simulink model "discrete"  (R2023b)
settings: Solver=FixedStepAuto  StartTime=0.0  StopTime=20  FixedStep=0.01  RelTol=1e-3
InitFcn:
  | clc;clear
  | close all
  | g = [0;2.092];
  | k1 = [-141.9203 -4.5243];
  | k2 = [-101.5134 -3.1941];
  | x0 = [0.4;-10];
libraries: simulink x1
settings Model: Creator=IHC  LastModifiedBy=IHC

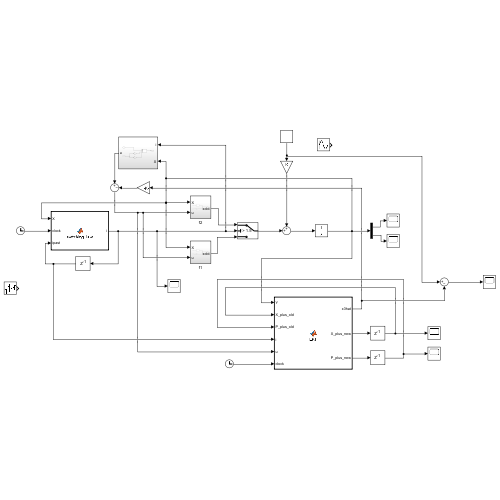
[thumbnail: Simulink's stored preview of the top-level diagram]
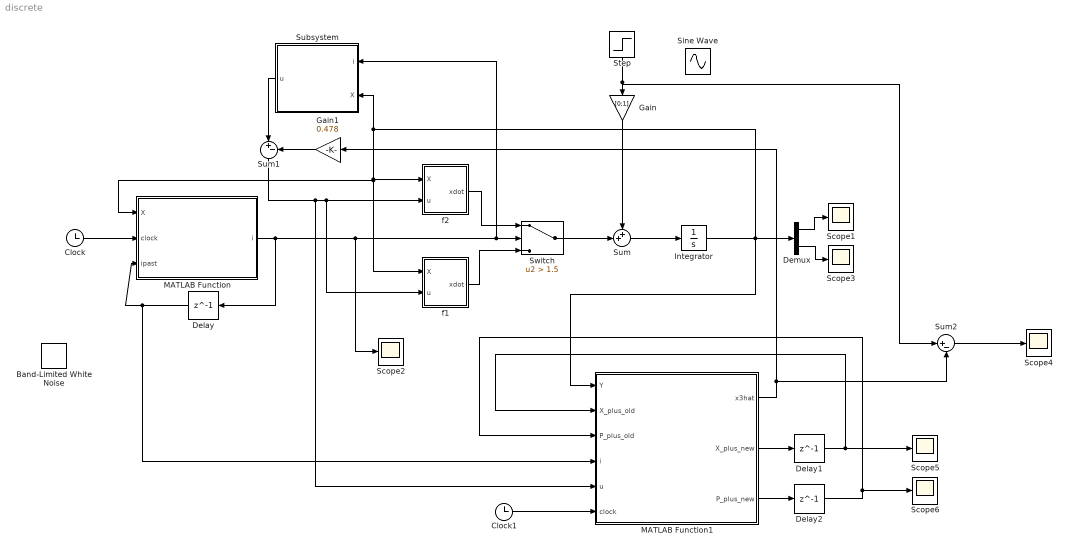
== system discrete ==
  Band-Limited White Noise : simulink/Sources/Band-Limited White Noise  Cov=[0.1]  Ts=0.1  seed=[23341]
  Clock : Clock
  Clock1 : Clock
  Delay : Delay  DelayLength=1  InitialCondition=2
  Delay1 : Delay  DelayLength=1  InitialCondition=[x0;0]
  Delay2 : Delay  DelayLength=1  InitialCondition=diag([0.001;0.001;10])
  Demux : Demux  Outputs=2
  Gain : Gain  Gain=[0;1]
  Gain1 : Gain  Gain=0.478
  Integrator : Integrator  InitialCondition=x0
  MATLAB Function : MATLAB Function  TreatAsAtomicUnit=on
  MATLAB Function1 : MATLAB Function  TreatAsAtomicUnit=on
  Scope{1..6} (6 alike) : Scope
  Sine Wave : Sin  SampleTime=0
  Step : Step  Time=0  SampleTime=0
  Subsystem : Subsystem
  Sum : Sum  Inputs=++|
  Sum1 : Sum  Inputs=|+-
  Sum2 : Sum  Inputs=|+-
  Switch : Switch  Criteria=u2 > Threshold  Threshold=1.5  SaturateOnIntegerOverflow=off  InputSameDT=off
  f1 : Subsystem
  f2 : Subsystem
  wires:
  Clock/1 -> MATLAB Function/2(clock)
  Subsystem/1(u) -> Sum1/1
  Demux/1 -> Scope1/1
  Demux/2 -> Scope3/1
  Delay/1 -> MATLAB Function1/4(i), MATLAB Function/3(ipast)
  MATLAB Function/1(i) -> Delay/1, Scope2/1, Subsystem/1(i), Switch/2
  f2/1(xdot) -> Switch/1
  f1/1(xdot) -> Switch/3
  Switch/1 -> Sum/2
  Sum/1 -> Integrator/1
  Gain/1 -> Sum/1
  Gain1/1 -> Sum1/2
  Step/1 -> Sum2/1, Gain/1
  Integrator/1 -> MATLAB Function1/1(Y), Demux/1, f1/1(X), MATLAB Function/1(X), f2/1(X), Subsystem/2(X)
  Sum1/1 -> MATLAB Function1/5(u), f1/2(u), f2/2(u)
  Clock1/1 -> MATLAB Function1/6(clock)
  MATLAB Function1/2(X_plus_new) -> Delay1/1
  MATLAB Function1/3(P_plus_new) -> Delay2/1
  Delay2/1 -> MATLAB Function1/3(P_plus_old), Scope6/1
  Delay1/1 -> Scope5/1, MATLAB Function1/2(X_plus_old)
  Sum2/1 -> Scope4/1
  MATLAB Function1/1(x3hat) -> Gain1/1, Sum2/2

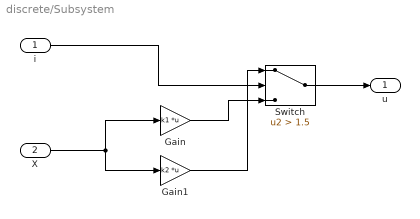
== system discrete/Subsystem ==
  i : Inport
  X : Inport  Port=2
  Gain : Gain  Gain=k1  Multiplication=Matrix(K*u)
  Gain1 : Gain  Gain=k2  Multiplication=Matrix(K*u)
  Switch : Switch  Criteria=u2 > Threshold  Threshold=1.5  SaturateOnIntegerOverflow=off  InputSameDT=off
  u : Outport
  wires:
  Switch/1 -> u/1
  i/1 -> Switch/2
  X/1 -> Gain1/1, Gain/1
  Gain/1 -> Switch/3
  Gain1/1 -> Switch/1

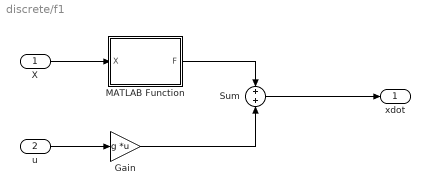
== system discrete/f1 ==
  X : Inport
  u : Inport  Port=2
  Gain : Gain  Gain=g  Multiplication=Matrix(K*u)
  MATLAB Function : MATLAB Function  TreatAsAtomicUnit=on
  Sum : Sum
  xdot : Outport
  wires:
  u/1 -> Gain/1
  X/1 -> MATLAB Function/1(X)
  Gain/1 -> Sum/2
  MATLAB Function/1(F) -> Sum/1
  Sum/1 -> xdot/1

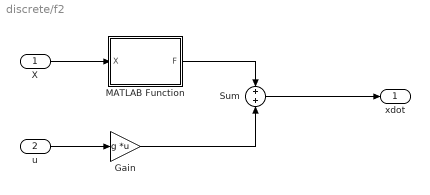
== system discrete/f2 ==
  X : Inport
  u : Inport  Port=2
  Gain : Gain  Gain=g  Multiplication=Matrix(K*u)
  MATLAB Function : MATLAB Function  TreatAsAtomicUnit=on
  Sum : Sum
  xdot : Outport
  wires:
  Sum/1 -> xdot/1
  u/1 -> Gain/1
  MATLAB Function/1(F) -> Sum/1
  Gain/1 -> Sum/2
  X/1 -> MATLAB Function/1(X)

== matlab function discrete/f2/MATLAB Function ==
  data: X input; F output
function F = fcn(X)
x1 = X(1);
x2 = X(2);
alpha = -7.2*10^10*(x1+0.5)*exp(-8750/(x2+350))+0.5;
beta = 1.506*10^13*(x1+0.5)*exp(-8750/(x2+350))-104.6;
f1=-2*x1+alpha;
f2 =-4.092*x2+beta;
F=[f1;f2];
end

== matlab function discrete/f1/MATLAB Function ==
  data: X input; F output
function F = fcn(X)
x1 = X(1);
x2 = X(2);
alpha = -7.2*10^10*(x1+0.5)*exp(-8750/(x2+350))+0.5;
beta = 1.506*10^13*(x1+0.5)*exp(-8750/(x2+350))-104.6;
f1=-0.5*x1+alpha;
f2 =-2.592*x2+beta;
F=[f1;f2];
end

== matlab function discrete/MATLAB Function ==
  data: X input; i output; clock input; ipast input
function i = switching_law(X,clock,ipast)
x1 = X(1);
x2 = X(2);
g = [0;2.092];
vx1 = zeros(1,2);
vx2 = zeros(1,2);

vx1(1,1) = [6175.531 135.679]*X;
vx1(1,2) = [135.679 4.3253]*X;
vx2(1,1) = [3590.3982 97.0491]*X;
vx2(1,2) = [97.0491 3.0536]*X;
alpha = -7.2*10^10*(x1+0.5)*exp(-8750/(x2+350))+0.5;
beta = 1.506*10^13*(x1+0.5)*exp(-8750/(x2+350))-104.6;
f1 = [-0.5*x1+alpha;-2.592*x2+beta];
f2 = [-2*x1+alpha;-4.092*x2+beta]; 
a = vx1*f1 - (1/4)*vx1*g*g'*vx1';
b = vx2*f2 - (1/4)*vx2*g*g'*vx2';

if mod(clock,0.1) == 0
    if b < a
        i = 2;
    else
        i = 1;
    end
else
    i = ipast;
end
end

== matlab function discrete/MATLAB Function1 ==
  data: Y input; X_plus_old input; P_plus_old input; i input; u input; x3hat output; clock input; X_plus_new output; P_plus_new output
function [x3hat,X_plus_new,P_plus_new]= EKF(Y,X_plus_old,P_plus_old,i,u,clock)
ts = 0.01;
H = [1 0 0;0 1 0];
M = eye(2);
L = ts*eye(3);
R = 1e-5*eye(2);
Q = diag([1,1,1]);
%extended Kalman filter
%time update
P_minus=Fd(X_plus_old,i,ts)*P_plus_old*Fd(X_plus_old,i,ts)'+L*Q*L';
x_minus=f(X_plus_old,u,i);
%measurment update
K = P_minus*H'*(H*P_minus*H'+M*R*M');
X_plus_new = x_minus+K*(Y-[x_minus(1);x_minus(2)]);
P_plus_new=(eye(3)-K*H)*P_minus;

x3hat = X_plus_old(3);




    function fc = f(X,i,u)
        x1 =X(1);x2 =X(2);x3=X(3);
        alpha = -7.2e10*(x1+0.5)*exp(-8750/(x2+350))+0.5;
        beta = 1.506e13*(x1+0.5)*exp(-8750/(x2+350))-104.6;
        f3 = 0;
        if i == 1
            f1 = -0.5*x1+alpha;
            f2 = -2.592*x2+beta+x3+2.092*u;
        elseif i == 2
            f1 = -2*x1+alpha;
            f2 = -4.092*x2+beta+x3+2.092*u;
        else
            f1 =x1+x2+x3+u;
            f2 =x1+x2+x3+u;
        end
        fc = [f1;f2;f3];
    end

    function fd = Fd(X,i,ts)
        x1 =X(1);x2 =X(2);x3=X(3);
        fd = [72000000000*exp(-8750/(x2 + 350)),-(8750*exp(-8750/(x2 + 350))*(72000000000*x1 + 36000000000))/(x2 + 350)^2, 0;
               15060000000000*exp(-8750/(x2 + 350)),(8750*exp(-8750/(x2 + 350))*(15060000000000*x1 + 7530000000000))/(x2 + 350)^2,1;
               0,0, 0];
        if i == 1
            fd = fd+[-0.5,0,0;0 -2.592 0;0 0 0];
        elseif i == 2
            fd = fd+[-2,0,0;0 -4.092 0;0 0 0];
        end
        fd = ts*fd+eye(3);
    end


end
